simulink model "TrajectoryFollowVehicle"  (R2024b)
settings: Solver=FixedStepAuto  StartTime=0  StopTime=1000  FixedStep=timeStep  RelTol=1e-3
PostLoadFcn:
  | load(fullfile(matlabroot,'toolbox','driving','drivingdata','rrScenarioSimTypes.mat'));
  | helperSLTrajectoryFollowerWithRRScenarioSetup
undefined symbols (not defined in the file or in its folder): Defined, Ego, Lane, lr, m, n, Pose, RRtimeStep, tau, tau2, timeStep, User, Velocity
libraries: roadrunnerscenario x6, simulink_extras x6, drivingvehiclecontroller x2, autolibshared x1
settings Model: Creator=The MathWorks, Inc.  LastModifiedBy=nobuakif
settings DataIOCC: SaveOutput=off  DSMLogging=off  InspectSignalLogs=on  SaveTime=off  ReturnWorkspaceOutputs=off
settings OptimizationCC: DefaultParameterBehavior=Inlined  ReuseModelBlockBuffer=off  ZeroExternalMemoryAtStartup=off  ZeroInternalMemoryAtStartup=off
settings DebuggingCC: ParameterTunabilityLossMsg=error  UnconnectedInputMsg=warning  UnconnectedOutputMsg=warning  UnconnectedLineMsg=warning
settings ModelReferenceCC: EnableRefExpFcnMdlSchedulingChecks=on  PropagateSignalLabelsOutOfModel=off
settings RTWCC: GenCodeOnly=on  GenerateReport=on  TargetLang=C++  GPUComputeCapability=3.5
settings CodeAppCC: ForceParamTrailComments=on
settings GRTTargetCC: TargetLangStandard=C++03 (ISO)  CodeInterfacePackaging=C++ class

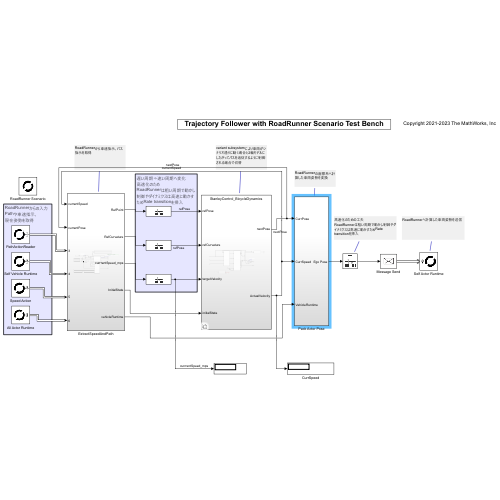
[thumbnail: Simulink's stored preview of the top-level diagram]
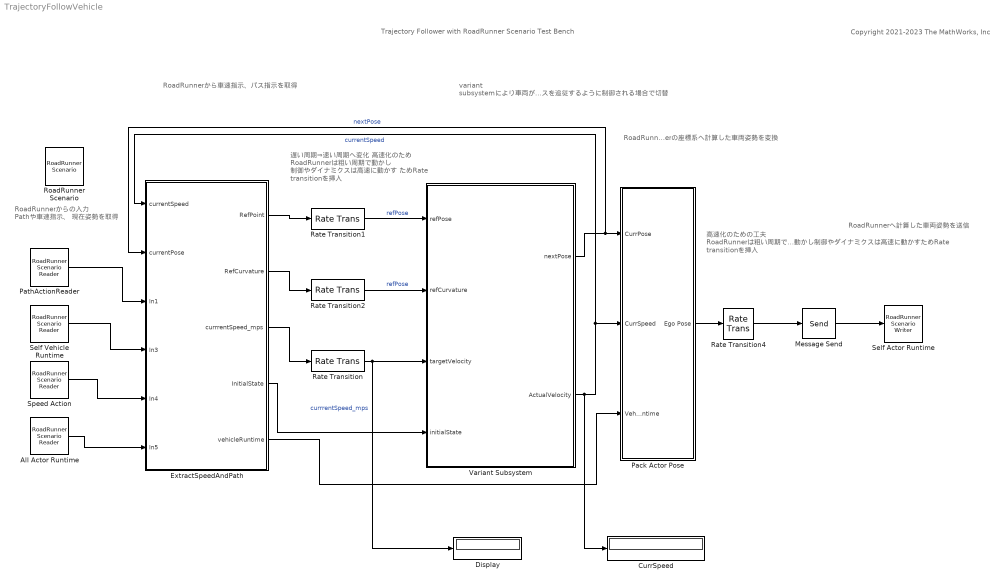
== system TrajectoryFollowVehicle ==
  note: 高速化のための工夫
      | RoadRunnerは粗い周期で動かし制御やダイナミクスは高速に動かすためRate transitionを挿入
  note: 遅い周期⇒速い周期へ変化
      | 高速化のため
      | RoadRunnerは粗い周期で動かし
      | 制御やダイナミクスは高速に動かす
      | ためRate transitionを挿入
  note: RoadRunnerからの入力
      | Pathや車速指示、
      | 現在姿勢を取得
  note: Trajectory Follower with RoadRunner Scenario Test Bench
  note: Copyright 2021-2023 The MathWorks, Inc
  note: RoadRunnerへ計算した車両姿勢を送信
  note: RoadRunnerの座標系へ計算した車両姿勢を変換
  note: variant subsystemにより車両がシナリオ通りに動く場合と2輪モデルにしたがってパスを追従するように制御される場合で切替
  note: RoadRunnerから車速指示、パス指示を取得
  All Actor Runtime : roadrunnerscenario/RoadRunner Scenario Reader  TopicCategory=Actor  ActorCategory=All Types  ActionType=Path Following  EventType=User-Defined  TopicType=Actor Pose  VehicleType=Vehicle Specifications  UserDefinedAction=Action1  UserDefinedEvent=Event1  Filter=None  SensorTopic=Target Poses  LaneBoundaryOutputTopic=Ego-Lane  SensorID=1  SampleTime=RRtimeStep
  CurrSpeed : Display
  Display : Display
  ExtractSpeedAndPath : Subsystem
  Message Send : Send  OutputPortMessageModes=m
  Pack Actor Pose : Subsystem
  PathActionReader : roadrunnerscenario/RoadRunner Scenario Reader  TopicCategory=Action  ActorCategory=Vehicle  ActionType=Path Following  EventType=User-Defined  TopicType=Actor Specifications  VehicleType=Vehicle Pose  UserDefinedAction=Action1  UserDefinedEvent=Event1  Filter=Self  SensorTopic=Target Poses  LaneBoundaryOutputTopic=Ego-Lane  SensorID=1  SampleTime=RRtimeStep
  Rate Transition : RateTransition  OutPortSampleTime=timeStep
  Rate Transition1 : RateTransition  OutPortSampleTime=timeStep
  Rate Transition2 : RateTransition  OutPortSampleTime=timeStep
  Rate Transition4 : RateTransition  OutPortSampleTime=RRtimeStep
  RoadRunner Scenario : roadrunnerscenario/RoadRunner Scenario  UserDefinedActions={}  UserDefinedEvents={}
  Self Actor Runtime : roadrunnerscenario/RoadRunner Scenario Writer  TopicCategory=Actor  ActorCategory=All Types  EventType=Action Complete  UserDefinedEvent=Event1  VehicleType=Vehicle Pose  TopicType=Actor Pose
  Self Vehicle Runtime : roadrunnerscenario/RoadRunner Scenario Reader  TopicCategory=Actor  ActorCategory=Vehicle  ActionType=Path Following  EventType=User-Defined  TopicType=Actor Specifications  VehicleType=Vehicle Pose  UserDefinedAction=Action1  UserDefinedEvent=Event1  Filter=Self  SensorTopic=Target Poses  LaneBoundaryOutputTopic=Ego-Lane  SensorID=1  SampleTime=RRtimeStep
  Speed Action : roadrunnerscenario/RoadRunner Scenario Reader  TopicCategory=Action  ActorCategory=All Types  ActionType=Speed Change  EventType=User-Defined  TopicType=Actor Specifications  VehicleType=Vehicle Specifications  UserDefinedAction=Action1  UserDefinedEvent=Event1  Filter=Self  SensorTopic=Target Poses  LaneBoundaryOutputTopic=Ego-Lane  SensorID=1  SampleTime=RRtimeStep
  Variant Subsystem : Subsystem  Variant=on
  wires:
  Rate Transition/1 -> Variant Subsystem/3(targetVelocity), Display/1  "currrentSpeed_mps"
  ExtractSpeedAndPath/5(vehicleRuntime) -> Pack Actor Pose/3(VehicleRuntime)
  Pack Actor Pose/1(Ego Pose) -> Rate Transition4/1
  Message Send/1 -> Self Actor Runtime/1
  Rate Transition4/1 -> Message Send/1
  Rate Transition1/1 -> Variant Subsystem/1(refPose)  "refPose"
  Variant Subsystem/2(ActualVelocity) -> CurrSpeed/1, ExtractSpeedAndPath/1(currentSpeed), Pack Actor Pose/2(CurrSpeed)  "currentSpeed"
  Variant Subsystem/1(nextPose) -> ExtractSpeedAndPath/2(currentPose), Pack Actor Pose/1(CurrPose)  "nextPose"
  Rate Transition2/1 -> Variant Subsystem/2(refCurvature)  "refPose"
  ExtractSpeedAndPath/4(InitialState) -> Variant Subsystem/4(initialState)
  PathActionReader/1 -> ExtractSpeedAndPath/3(In1)
  Self Vehicle Runtime/1 -> ExtractSpeedAndPath/4(In3)
  Speed Action/1 -> ExtractSpeedAndPath/5(In4)
  All Actor Runtime/1 -> ExtractSpeedAndPath/6(In5)
  ExtractSpeedAndPath/1(RefPoint) -> Rate Transition1/1
  ExtractSpeedAndPath/2(RefCurvature) -> Rate Transition2/1
  ExtractSpeedAndPath/3(currrentSpeed_mps) -> Rate Transition/1

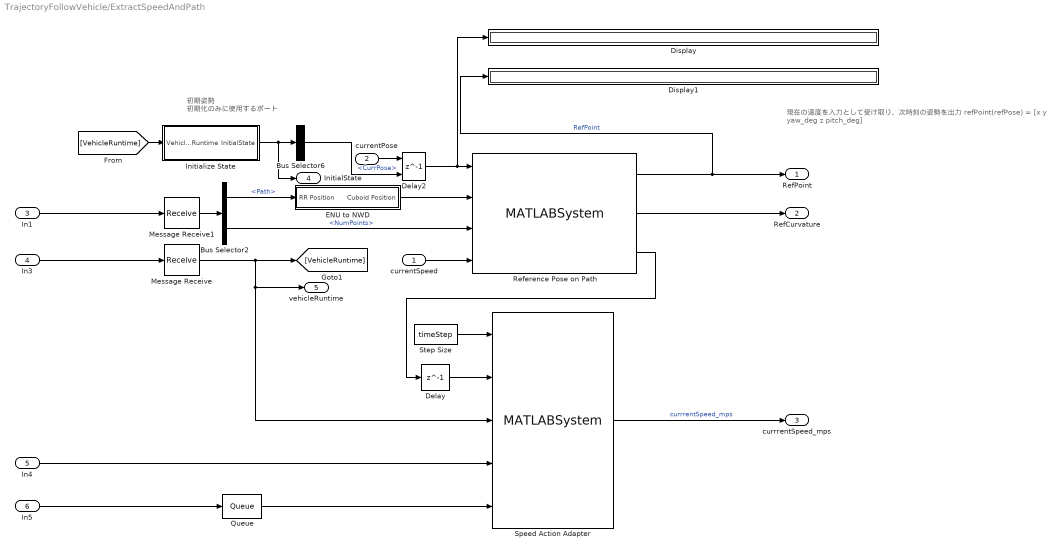
== system TrajectoryFollowVehicle/ExtractSpeedAndPath ==
  note: 現在の速度を入力として受け取り、次時刻の姿勢を出力
      | refPoint(refPose) = [x y yaw_deg z pitch_deg]
  note: 初期姿勢
      | 初期化のみに使用するポート
  currentSpeed : Inport
  currentPose : Inport  Port=2
  In1 : Inport  Port=3
  In3 : Inport  Port=4
  In4 : Inport  Port=5
  In5 : Inport  Port=6
  Bus Selector2 : BusSelector  OutputSignals=PathTarget.Path,PathTarget.NumPoints
  Bus Selector6 : BusSelector  OutputSignals=CurrPose
  Delay : Delay  DelayLength=1  InitialCondition=logical(0)
  Delay2 : Delay  DelayLength=1  InitialConditionSource=Input port
      settings: InputPortMap=u0,p4
  Display : Display
  Display1 : Display
  ENU to NWD : Subsystem
  Initialize State : Subsystem
  Message Receive : Receive  InputPortMessageModes=m
  Message Receive1 : Receive  InputPortMessageModes=m
  Queue : Queue  InputPortMessageModes=m  OutputPortMessageModes=m  OverwriteOldest=on  Capacity=16  QueueType=LIFO
  Reference Pose on Path : MATLABSystem  System=HelperReferencePoseOnPath  timeStep=timeStep  vehicleOnPath=useDynamicsStanley == false  long_offset=lf  debugFig=false  searchIndx=10
      mask Type: HelperReferencePoseOnPath
      mask Display:
      | disp(['HelperReferencePoseOnPath' char(10) '' char(10) '' char(10) '' char(10) '']);
      | port_label('input',1,'PrevVehicleInfo');
      | port_label('input',2,'Trajectory');
      | port_label('input',3,'NumTrajPoints');
      | port_label('input',4,'currentSpeed');
      | port_label('output',1,'RefPointOnPath');
      | port_label('output',2,'RefCurvature');
      | port_label('output',3,'IsGoalReached');
  Speed Action Adapter : MATLABSystem  InputPortMessageModes=n,n,n,m,m  System=HelperSpeedActionAdapter
      mask Type: HelperSpeedActionAdapter
      mask Display:
      | disp(['HelperSpeedActionAdapter' char(10) '' char(10) '']);
      | port_label('input',1,'timestep');
      | port_label('input',2,'stopVehicle');
      | port_label('input',3,'vehicleRuntime');
      | port_label('input',4,'msgSpeedAction');
      | port_label('input',5,'msgAllVehicleRuntime');
      | port_label('output',1,'currentSpeed');
  Step Size : Constant  Value=timeStep
  RefPoint : Outport
  RefCurvature : Outport  Port=2
  currrentSpeed_mps : Outport  Port=3
  InitialState : Outport  Port=4
  vehicleRuntime : Outport  Port=5
  wires:
  Bus Selector6/1 -> Delay2/2  "<CurrPose>"
  Delay/1 -> Speed Action Adapter/2
  Reference Pose on Path/1 -> Display1/1, RefPoint/1  "RefPoint"
  Step Size/1 -> Speed Action Adapter/1
  [VehicleRuntime] -> Initialize State/1(VehicleRuntime)
  Message Receive1/1 -> Bus Selector2/1
  Initialize State/1(InitialState) -> InitialState/1, Bus Selector6/1
  Reference Pose on Path/3 -> Delay/1
  Bus Selector2/1 -> ENU to NWD/1(RR Position)  "<Path>"
  Message Receive/1 -> Speed Action Adapter/3, vehicleRuntime/1, [VehicleRuntime]
  In4/1 -> Speed Action Adapter/4
  ENU to NWD/1(Cuboid Position) -> Reference Pose on Path/2
  Bus Selector2/2 -> Reference Pose on Path/3  "<NumPoints>"
  In3/1 -> Message Receive/1
  Reference Pose on Path/2 -> RefCurvature/1
  In5/1 -> Queue/1
  Speed Action Adapter/1 -> currrentSpeed_mps/1  "currrentSpeed_mps"
  In1/1 -> Message Receive1/1
  currentSpeed/1 -> Reference Pose on Path/4
  Queue/1 -> Speed Action Adapter/5
  Delay2/1 -> Display/1, Reference Pose on Path/1
  currentPose/1 -> Delay2/1

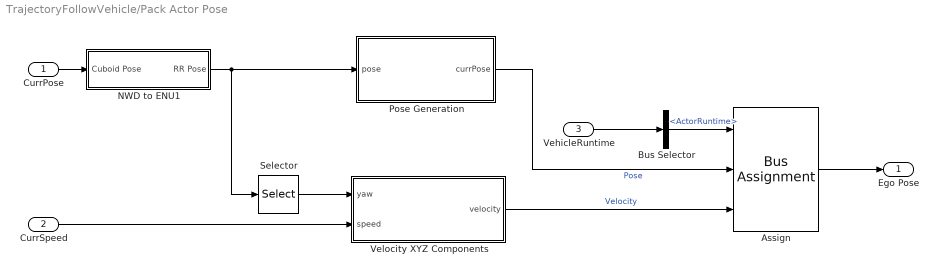
== system TrajectoryFollowVehicle/Pack Actor Pose ==
  CurrPose : Inport
  CurrSpeed : Inport  Port=2
  VehicleRuntime : Inport  Port=3
  Assign : BusAssignment  AssignedSignals=Pose,Velocity
  Bus Selector : BusSelector  OutputSignals=ActorRuntime
  NWD to ENU1 : Subsystem
  Pose Generation : MATLAB Function  TreatAsAtomicUnit=on
  Selector : Selector  InputPortWidth=5  IndexOptions=Index vector (dialog)  Indices=3  OutputSizes=1
  Velocity XYZ Components : MATLAB Function  TreatAsAtomicUnit=on
  Ego Pose : Outport
  wires:
  Velocity XYZ Components/1(velocity) -> Assign/3  "Velocity"
  Pose Generation/1(currPose) -> Assign/2  "Pose"
  CurrPose/1 -> NWD to ENU1/1(Cuboid Pose)
  Selector/1 -> Velocity XYZ Components/1(yaw)
  CurrSpeed/1 -> Velocity XYZ Components/2(speed)
  VehicleRuntime/1 -> Bus Selector/1
  Bus Selector/1 -> Assign/1  "<ActorRuntime>"
  Assign/1 -> Ego Pose/1
  NWD to ENU1/1(RR Pose) -> Selector/1, Pose Generation/1(pose)

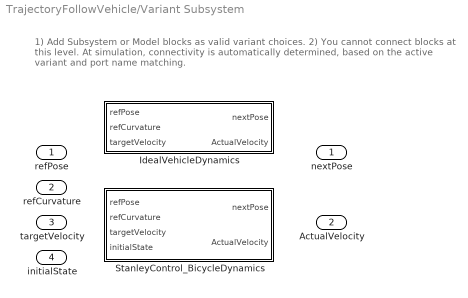
== system TrajectoryFollowVehicle/Variant Subsystem ==
  note: 1) Add Subsystem or Model blocks as valid variant choices.
      | 2) You cannot connect blocks at this level. At simulation, connectivity is automatically
      | determined, based on the active variant and port name matching.
  refPose : Inport
  refCurvature : Inport  Port=2
  targetVelocity : Inport  Port=3
  initialState : Inport  Port=4
  IdealVehicleDynamics : Subsystem  VariantControl=useDynamicsStanley == false
  StanleyControl_BicycleDynamics : Subsystem  VariantControl=useDynamicsStanley == true
  nextPose : Outport
  ActualVelocity : Outport  Port=2

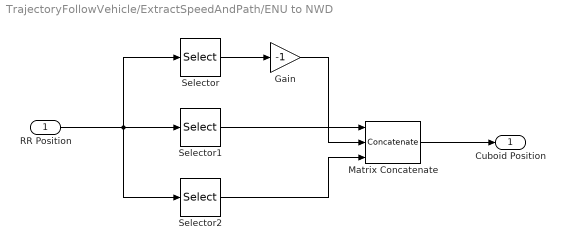
== system TrajectoryFollowVehicle/ExtractSpeedAndPath/ENU to NWD ==
  RR Position : Inport
  Gain : Gain  Gain=-1
  Matrix Concatenate : Concatenate  NumInputs=3  Mode=Multidimensional array  ConcatenateDimension=2
  Selector : Selector  NumberOfDimensions=2  InputPortWidth=3  IndexOptions=Select all,Index vector (dialog)  Indices=[1 3],1  OutputSizes=1,1
  Selector1 : Selector  NumberOfDimensions=2  InputPortWidth=3  IndexOptions=Select all,Index vector (dialog)  Indices=[1 3],2  OutputSizes=1,1
  Selector2 : Selector  NumberOfDimensions=2  InputPortWidth=3  IndexOptions=Select all,Index vector (dialog)  Indices=[1 3],3  OutputSizes=1,1
  Cuboid Position : Outport
  wires:
  Gain/1 -> Matrix Concatenate/2
  Selector1/1 -> Matrix Concatenate/1
  Selector2/1 -> Matrix Concatenate/3
  Selector/1 -> Gain/1
  RR Position/1 -> Selector/1, Selector1/1, Selector2/1
  Matrix Concatenate/1 -> Cuboid Position/1

== system TrajectoryFollowVehicle/ExtractSpeedAndPath/Initialize State ==
  VehicleRuntime : Inport
  Calculate Initial States : Subsystem
  Constant : Constant  Value=0
  Delay : Delay  DelayLength=1  InitialCondition=1
  InitialState : Outport
  wires:
  Delay/1 -> Calculate Initial States/Trigger
  Constant/1 -> Delay/1
  Calculate Initial States/1(EgoInitialState) -> InitialState/1
  VehicleRuntime/1 -> Calculate Initial States/1(EgoRuntime)

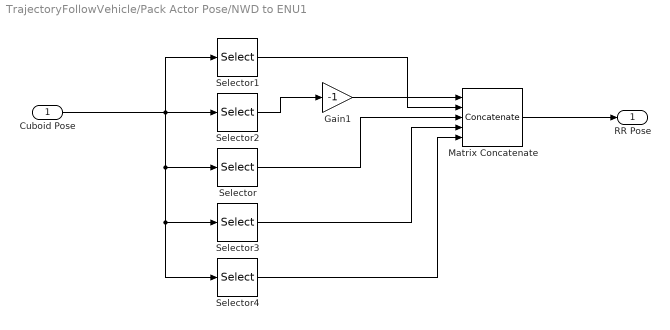
== system TrajectoryFollowVehicle/Pack Actor Pose/NWD to ENU1 ==
  Cuboid Pose : Inport
  Gain1 : Gain  Gain=-1
  Matrix Concatenate : Concatenate  NumInputs=5  Mode=Multidimensional array  ConcatenateDimension=2
  Selector : Selector  InputPortWidth=5  IndexOptions=Index vector (dialog)  Indices=3  OutputSizes=1
  Selector1 : Selector  InputPortWidth=5  IndexOptions=Index vector (dialog)  Indices=1  OutputSizes=1
  Selector2 : Selector  InputPortWidth=5  IndexOptions=Index vector (dialog)  Indices=2  OutputSizes=1
  Selector3 : Selector  InputPortWidth=5  IndexOptions=Index vector (dialog)  Indices=4  OutputSizes=1
  Selector4 : Selector  InputPortWidth=5  IndexOptions=Index vector (dialog)  Indices=5  OutputSizes=1
  RR Pose : Outport
  wires:
  Gain1/1 -> Matrix Concatenate/1
  Cuboid Pose/1 -> Selector2/1, Selector/1, Selector3/1, Selector4/1, Selector1/1
  Selector/1 -> Matrix Concatenate/3
  Selector1/1 -> Matrix Concatenate/2
  Selector2/1 -> Gain1/1
  Matrix Concatenate/1 -> RR Pose/1
  Selector3/1 -> Matrix Concatenate/4
  Selector4/1 -> Matrix Concatenate/5

== system TrajectoryFollowVehicle/Variant Subsystem/IdealVehicleDynamics ==
  refPose : Inport
  refCurvature : Inport  Port=2
  targetVelocity : Inport  Port=3
  Terminator : Terminator
  nextPose : Outport
  ActualVelocity : Outport  Port=2
  wires:
  targetVelocity/1 -> ActualVelocity/1
  refCurvature/1 -> Terminator/1
  refPose/1 -> nextPose/1

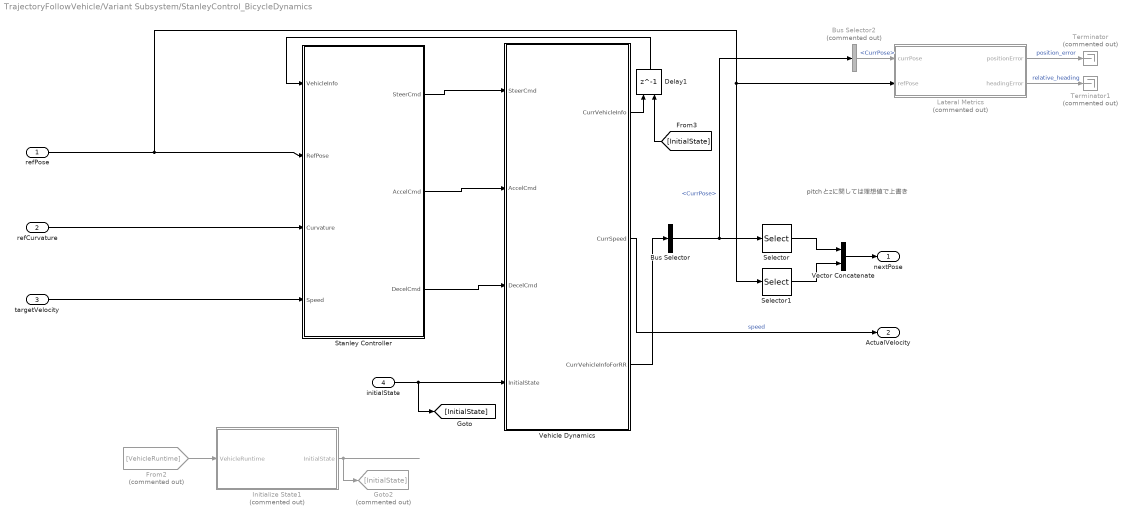
== system TrajectoryFollowVehicle/Variant Subsystem/StanleyControl_BicycleDynamics ==
  note: pitchとzに関しては理想値で上書き
  refPose : Inport
  refCurvature : Inport  Port=2
  targetVelocity : Inport  Port=3
  initialState : Inport  Port=4
  Bus Selector : BusSelector  OutputSignals=CurrPose
  Bus Selector2 : BusSelector  Commented=on  OutputSignals=CurrPose
  Delay1 : Delay  DelayLength=1  InitialConditionSource=Input port
      settings: InputPortMap=u0,p4
  From2 : From  Commented=on  GotoTag=VehicleRuntime
  Goto2 : Goto  Commented=on  GotoTag=InitialState
  Initialize State1 : Subsystem  Commented=on
  Lateral Metrics : MATLAB Function  Commented=on  TreatAsAtomicUnit=on
  Selector : Selector  InputPortWidth=5  IndexOptions=Index vector (dialog)  Indices=1:3  OutputSizes=1
  Selector1 : Selector  InputPortWidth=5  IndexOptions=Index vector (dialog)  Indices=4:5  OutputSizes=1
  Stanley Controller : Subsystem
  Terminator : Terminator  Commented=on
  Terminator1 : Terminator  Commented=on
  Vector Concatenate : Concatenate
  Vehicle Dynamics : Subsystem
  nextPose : Outport
  ActualVelocity : Outport  Port=2
  wires:
  Stanley Controller/3(DecelCmd) -> Vehicle Dynamics/3(DecelCmd)
  Vehicle Dynamics/1(CurrVehicleInfo) -> Delay1/1
  refCurvature/1 -> Stanley Controller/3(Curvature)
  Vehicle Dynamics/2(CurrSpeed) -> ActualVelocity/1  "speed"
  Delay1/1 -> Stanley Controller/1(VehicleInfo)
  Stanley Controller/1(SteerCmd) -> Vehicle Dynamics/1(SteerCmd)
  targetVelocity/1 -> Stanley Controller/4(Speed)
  Bus Selector/1 -> Bus Selector2/1, Selector/1  "<CurrPose>"
  Stanley Controller/2(AccelCmd) -> Vehicle Dynamics/2(AccelCmd)
  [InitialState] -> Delay1/2
  Initialize State1/1(InitialState) -> Goto2/1
  From2/1 -> Initialize State1/1(VehicleRuntime)
  initialState/1 -> [InitialState], Vehicle Dynamics/4(InitialState)
  Selector/1 -> Vector Concatenate/1
  Selector1/1 -> Vector Concatenate/2
  Vector Concatenate/1 -> nextPose/1
  refPose/1 -> Selector1/1, Lateral Metrics/2(refPose), Stanley Controller/2(RefPose)
  Lateral Metrics/2(headingError) -> Terminator1/1  "relative_heading"
  Bus Selector2/1 -> Lateral Metrics/1(currPose)  "<CurrPose>"
  Lateral Metrics/1(positionError) -> Terminator/1  "position_error"
  Vehicle Dynamics/3(CurrVehicleInfoForRR) -> Bus Selector/1

== system TrajectoryFollowVehicle/ExtractSpeedAndPath/Initialize State/Calculate Initial States ==
  EgoRuntime : Inport
  Trigger : TriggerPort  VariantControl=(inherit)  InitialTriggerSignalState=negative  PortDimensions=1
  Calculate Initial States : MATLAB Function  TreatAsAtomicUnit=on
  EgoInitialState : Outport
  wires:
  EgoRuntime/1 -> Calculate Initial States/1(egoRuntime)
  Calculate Initial States/1(egoInitialState) -> EgoInitialState/1

== system TrajectoryFollowVehicle/Variant Subsystem/StanleyControl_BicycleDynamics/Initialize State1 ==
  VehicleRuntime : Inport
  Calculate Initial States : Subsystem
  Constant : Constant  Value=0
  Delay : Delay  DelayLength=1  InitialCondition=1
  InitialState : Outport
  wires:
  Delay/1 -> Calculate Initial States/Trigger
  Constant/1 -> Delay/1
  Calculate Initial States/1(EgoInitialState) -> InitialState/1
  VehicleRuntime/1 -> Calculate Initial States/1(EgoRuntime)

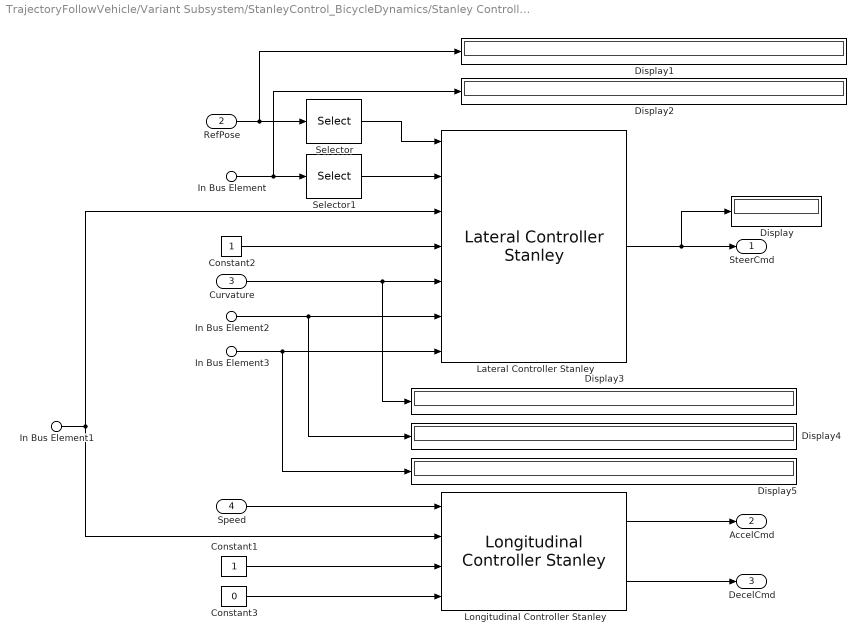
== system TrajectoryFollowVehicle/Variant Subsystem/StanleyControl_BicycleDynamics/Stanley Controller ==
  In Bus Element : Inport  PortName=VehicleInfo  Element=CurrPose
  In Bus Element1 : Inport  PortName=VehicleInfo  Element=CurrVelocity
  In Bus Element2 : Inport  PortName=VehicleInfo  Element=CurrYawRate
  In Bus Element3 : Inport  PortName=VehicleInfo  Element=CurrSteer
  RefPose : Inport  Port=2
  Curvature : Inport  Port=3
  Speed : Inport  Port=4
  Constant1 : Constant
  Constant2 : Constant
  Constant3 : Constant  Value=0
  Display{,1..5} (6 alike) : Display
  Lateral Controller Stanley : drivingvehiclecontroller/Lateral Controller Stanley  ModelType=Dynamic bicycle model  PositionGainF=3  PositionGainR=2.5  YawRateGain=0.2  DelayGain=0.2  VehicleMass=m  Lf=lf  Lr=lr  TireStiffness=Cf  Wheelbase=2.8  MaxSteeringAngle=30
  Longitudinal Controller Stanley : drivingvehiclecontroller/Longitudinal Controller Stanley  Kp=2  Ki=1  SampleTime=timeStep  MaxAcceleration=max_ac  MaxDeceleration=max_dc
  Selector : Selector  InputPortWidth=5  IndexOptions=Index vector (dialog)  Indices=[1:3]  OutputSizes=1
  Selector1 : Selector  InputPortWidth=5  IndexOptions=Index vector (dialog)  Indices=[1:3]  OutputSizes=1
  SteerCmd : Outport
  AccelCmd : Outport  Port=2
  DecelCmd : Outport  Port=3
  wires:
  In Bus Element/1 -> Display2/1, Selector1/1
  Lateral Controller Stanley/1 -> Display/1, SteerCmd/1
  In Bus Element2/1 -> Display4/1, Lateral Controller Stanley/6
  In Bus Element1/1 -> Lateral Controller Stanley/3, Longitudinal Controller Stanley/2
  Constant1/1 -> Longitudinal Controller Stanley/3
  Longitudinal Controller Stanley/2 -> DecelCmd/1
  Constant2/1 -> Lateral Controller Stanley/4
  In Bus Element3/1 -> Display5/1, Lateral Controller Stanley/7
  Constant3/1 -> Longitudinal Controller Stanley/4
  RefPose/1 -> Display1/1, Selector/1
  Longitudinal Controller Stanley/1 -> AccelCmd/1
  Curvature/1 -> Display3/1, Lateral Controller Stanley/5
  Speed/1 -> Longitudinal Controller Stanley/1
  Selector/1 -> Lateral Controller Stanley/1
  Selector1/1 -> Lateral Controller Stanley/2

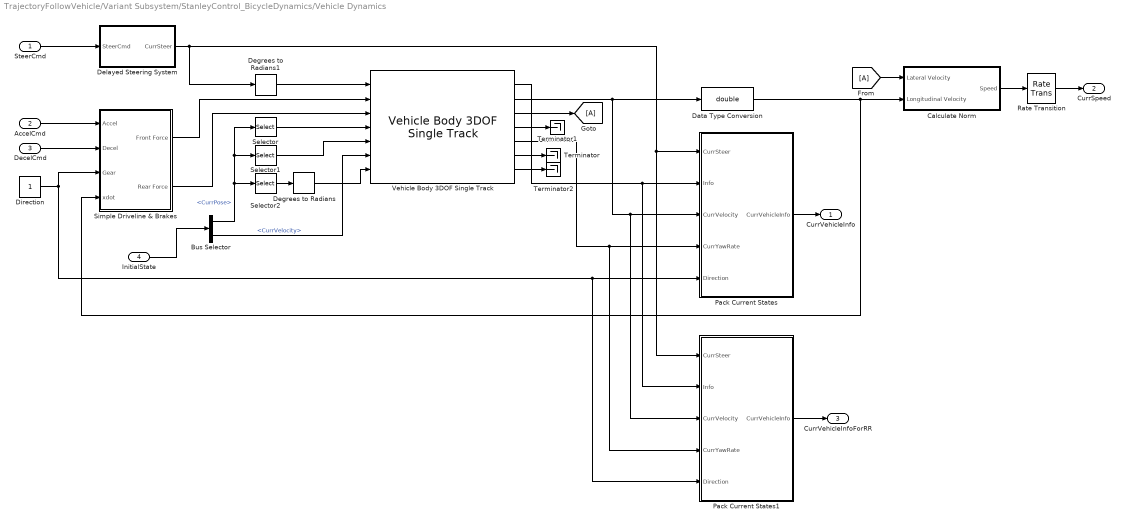
== system TrajectoryFollowVehicle/Variant Subsystem/StanleyControl_BicycleDynamics/Vehicle Dynamics ==
  SteerCmd : Inport
  AccelCmd : Inport  Port=2
  DecelCmd : Inport  Port=3
  InitialState : Inport  Port=4
  Bus Selector : BusSelector  OutputSignals=CurrPose,CurrVelocity
  Calculate Norm : Subsystem
  Data Type Conversion : DataTypeConversion  OutDataTypeStr=double  SaturateOnIntegerOverflow=off  RndMeth=Floor
  Degrees to Radians : simulink_extras/Transformations/Degrees to Radians
  Degrees to Radians1 : simulink_extras/Transformations/Degrees to Radians
  Delayed Steering System : Subsystem
  Direction : Constant
  From : From
  Goto : Goto
  Pack Current States : Subsystem
  Pack Current States1 : Subsystem
  Rate Transition : RateTransition
  Selector : Selector  InputPortWidth=5  IndexOptions=Index vector (dialog)  Indices=1  OutputSizes=1
  Selector1 : Selector  InputPortWidth=5  IndexOptions=Index vector (dialog)  Indices=2  OutputSizes=1
  Selector2 : Selector  InputPortWidth=5  IndexOptions=Index vector (dialog)  Indices=3  OutputSizes=1
  Simple Driveline & Brakes : Subsystem
  Terminator : Terminator
  Terminator1 : Terminator
  Terminator2 : Terminator
  Vehicle Body 3DOF Single Track : autolibshared/Vehicle Body 3DOF Single Track  trackMode=Single (bicycle)  inputMode=External longitudinal forces  frontSteerMode=on  rearSteerMode=off  windMode=off  muMode=off  extFMode=off  extMMode=off  htchFMode=off  htchMMode=off  extXo=on  extpsio=on  extxdoto=on  extro=off  extYo=on  extTamb=off  extydoto=off  aMode=2  NF=2  NR=2  m=m  a=lf  b=lr  h=0.35  dh=1  hh=0.2  X_o=0  xdot_o=0  CalphaMode=off  sigmaMode=off  d=0  hl=0  w=[1.4,1.4]  Cy_f=Cf  Cy_r=Cr  sigma_f=.1  sigma_r=.1  alpha_f_brk=[-.1 .1]  Cy_f_data=[-9e3 9e3]  alpha_r_brk=[-.1 .1]  Cy_r_data=[-9e3 9e3]  Y_o=0  ydot_o=0  Izz=Iz  psi_o=0  r_o=0  Af=0  Cd=.3  Cl=.1  Cpm=.1  beta_w=[0:0.01:0.3]  Cs=[0:0.03:0.9]  Cym=[0:0.01:0.3]  Pabs=101325  Tair=273  g=9.81  mu=1  xdot_tol=.01  Fznom=5000  Fxtire_sat=7e4  Fytire_sat=7e4  longOff=0  latOff=0  vertOff=0  wrapAng=off
  CurrVehicleInfo : Outport  VectorParamsAs1DForOutWhenUnconnected=off
  CurrSpeed : Outport  Port=2
  CurrVehicleInfoForRR : Outport  Port=3  VectorParamsAs1DForOutWhenUnconnected=off
  wires:
  DecelCmd/1 -> Simple Driveline & Brakes/2(Decel)
  AccelCmd/1 -> Simple Driveline & Brakes/1(Accel)
  SteerCmd/1 -> Delayed Steering System/1(SteerCmd)
  Direction/1 -> Pack Current States1/5(Direction), Pack Current States/5(Direction), Simple Driveline & Brakes/3(Gear)
  Vehicle Body 3DOF Single Track/2 -> Data Type Conversion/1, Pack Current States1/3(CurrVelocity), Pack Current States/3(CurrVelocity)
  Delayed Steering System/1(CurrSteer) -> Degrees to Radians1/1, Pack Current States1/1(CurrSteer), Pack Current States/1(CurrSteer)
  From/1 -> Calculate Norm/1(Lateral Velocity)
  Calculate Norm/1(Speed) -> Rate Transition/1
  Vehicle Body 3DOF Single Track/1 -> Pack Current States1/2(Info), Pack Current States/2(Info)
  Vehicle Body 3DOF Single Track/4 -> Terminator1/1
  Vehicle Body 3DOF Single Track/5 -> Pack Current States1/4(CurrYawRate), Pack Current States/4(CurrYawRate)
  Pack Current States/1(CurrVehicleInfo) -> CurrVehicleInfo/1
  Vehicle Body 3DOF Single Track/3 -> Goto/1
  Data Type Conversion/1 -> Calculate Norm/2(Longitudinal Velocity), Simple Driveline & Brakes/4(xdot)
  Rate Transition/1 -> CurrSpeed/1
  Vehicle Body 3DOF Single Track/7 -> Terminator2/1
  Vehicle Body 3DOF Single Track/6 -> Terminator/1
  InitialState/1 -> Bus Selector/1
  Degrees to Radians1/1 -> Vehicle Body 3DOF Single Track/1
  Simple Driveline & Brakes/1(Front Force) -> Vehicle Body 3DOF Single Track/2
  Simple Driveline & Brakes/2(Rear Force) -> Vehicle Body 3DOF Single Track/3
  Bus Selector/1 -> Selector2/1, Selector1/1, Selector/1  "<CurrPose>"
  Selector/1 -> Vehicle Body 3DOF Single Track/4
  Selector1/1 -> Vehicle Body 3DOF Single Track/5
  Selector2/1 -> Degrees to Radians/1
  Bus Selector/2 -> Vehicle Body 3DOF Single Track/6  "<CurrVelocity>"
  Degrees to Radians/1 -> Vehicle Body 3DOF Single Track/7
  Pack Current States1/1(CurrVehicleInfo) -> CurrVehicleInfoForRR/1

== system TrajectoryFollowVehicle/Variant Subsystem/StanleyControl_BicycleDynamics/Initialize State1/Calculate Initial States ==
  EgoRuntime : Inport
  Trigger : TriggerPort  VariantControl=(inherit)  InitialTriggerSignalState=negative  PortDimensions=1
  Calculate Initial States : MATLAB Function  TreatAsAtomicUnit=on
  EgoInitialState : Outport
  wires:
  EgoRuntime/1 -> Calculate Initial States/1(egoRuntime)
  Calculate Initial States/1(egoInitialState) -> EgoInitialState/1

== system TrajectoryFollowVehicle/Variant Subsystem/StanleyControl_BicycleDynamics/Vehicle Dynamics/Calculate Norm ==
  Lateral Velocity : Inport
  Longitudinal Velocity : Inport  Port=2
  Add : Sum
  Math Function : Math  Operator=square
  Math Function1 : Math  Operator=square
  Sqrt : Sqrt
  Speed : Outport
  wires:
  Add/1 -> Sqrt/1
  Math Function1/1 -> Add/2
  Math Function/1 -> Add/1
  Sqrt/1 -> Speed/1
  Lateral Velocity/1 -> Math Function/1
  Longitudinal Velocity/1 -> Math Function1/1

== system TrajectoryFollowVehicle/Variant Subsystem/StanleyControl_BicycleDynamics/Vehicle Dynamics/Delayed Steering System ==
  SteerCmd : Inport
  Add : Sum  Inputs=+-
  Delay : TransferFcn  Denominator=[0.1 0]
  Display : Display
  Display1 : Display
  Display2 : Display
  CurrSteer : Outport  VectorParamsAs1DForOutWhenUnconnected=off
  wires:
  Add/1 -> Display/1, Delay/1
  SteerCmd/1 -> Display2/1, Add/1
  Delay/1 -> Display1/1, Add/2, CurrSteer/1

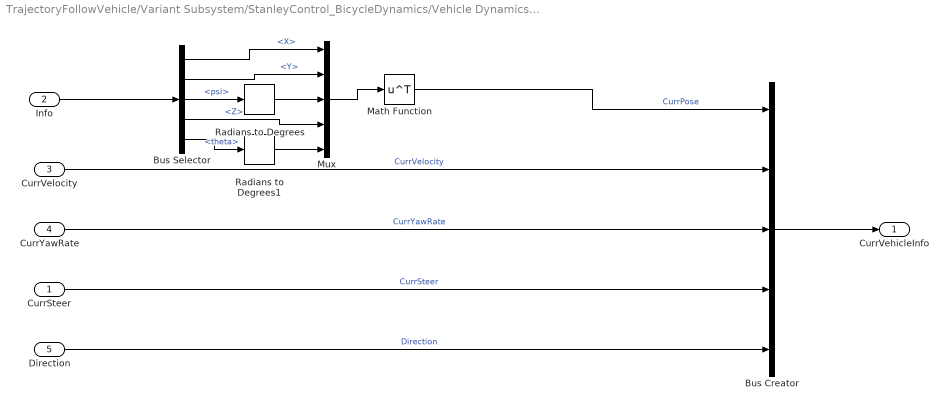
== system TrajectoryFollowVehicle/Variant Subsystem/StanleyControl_BicycleDynamics/Vehicle Dynamics/Pack Current States ==
  CurrSteer : Inport
  Info : Inport  Port=2
  CurrVelocity : Inport  Port=3
  CurrYawRate : Inport  Port=4
  Direction : Inport  Port=5
  Bus Creator : BusCreator  Inputs=5  OutDataTypeStr=Bus: BusVehicleInfo  NonVirtualBus=on
      settings: InheritFromInputs=off
  Bus Selector : BusSelector  OutputSignals=InertFrm.RearAxl.Disp.X,InertFrm.RearAxl.Disp.Y,InertFrm.Cg.Ang.psi,InertFrm.RearAxl.Disp.Z,InertFrm.Cg.Ang.theta
  Math Function : Math  Operator=transpose  SignedPower=on
  Mux : Mux  Inputs=5
  Radians to Degrees : simulink_extras/Transformations/Radians to Degrees
  Radians to Degrees1 : simulink_extras/Transformations/Radians to Degrees
  CurrVehicleInfo : Outport  VectorParamsAs1DForOutWhenUnconnected=off
  wires:
  CurrVelocity/1 -> Bus Creator/2  "CurrVelocity"
  CurrSteer/1 -> Bus Creator/4  "CurrSteer"
  Math Function/1 -> Bus Creator/1  "CurrPose"
  CurrYawRate/1 -> Bus Creator/3  "CurrYawRate"
  Direction/1 -> Bus Creator/5  "Direction"
  Mux/1 -> Math Function/1
  Info/1 -> Bus Selector/1
  Radians to Degrees/1 -> Mux/3
  Bus Selector/2 -> Mux/2  "<Y>"
  Bus Selector/1 -> Mux/1  "<X>"
  Bus Selector/3 -> Radians to Degrees/1  "<psi>"
  Bus Creator/1 -> CurrVehicleInfo/1
  Bus Selector/4 -> Mux/4  "<Z>"
  Bus Selector/5 -> Radians to Degrees1/1  "<theta>"
  Radians to Degrees1/1 -> Mux/5

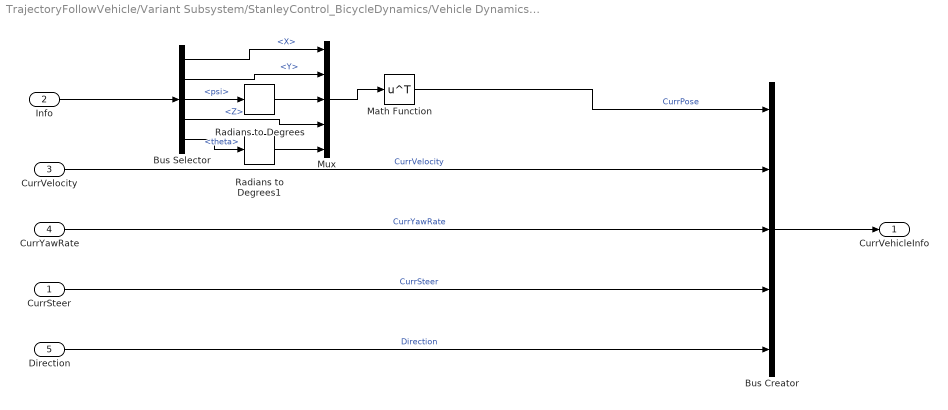
== system TrajectoryFollowVehicle/Variant Subsystem/StanleyControl_BicycleDynamics/Vehicle Dynamics/Pack Current States1 ==
  CurrSteer : Inport
  Info : Inport  Port=2
  CurrVelocity : Inport  Port=3
  CurrYawRate : Inport  Port=4
  Direction : Inport  Port=5
  Bus Creator : BusCreator  Inputs=5  OutDataTypeStr=Bus: BusVehicleInfo  NonVirtualBus=on
      settings: InheritFromInputs=off
  Bus Selector : BusSelector  OutputSignals=InertFrm.Cg.Disp.X,InertFrm.Cg.Disp.Y,InertFrm.Cg.Ang.psi,InertFrm.Cg.Disp.Z,InertFrm.Cg.Ang.theta
  Math Function : Math  Operator=transpose  SignedPower=on
  Mux : Mux  Inputs=5
  Radians to Degrees : simulink_extras/Transformations/Radians to Degrees
  Radians to Degrees1 : simulink_extras/Transformations/Radians to Degrees
  CurrVehicleInfo : Outport  VectorParamsAs1DForOutWhenUnconnected=off
  wires:
  Radians to Degrees1/1 -> Mux/5
  Bus Selector/5 -> Radians to Degrees1/1  "<theta>"
  Bus Selector/4 -> Mux/4  "<Z>"
  Bus Creator/1 -> CurrVehicleInfo/1
  Bus Selector/3 -> Radians to Degrees/1  "<psi>"
  Bus Selector/1 -> Mux/1  "<X>"
  Bus Selector/2 -> Mux/2  "<Y>"
  Radians to Degrees/1 -> Mux/3
  Info/1 -> Bus Selector/1
  Mux/1 -> Math Function/1
  Direction/1 -> Bus Creator/5  "Direction"
  CurrYawRate/1 -> Bus Creator/3  "CurrYawRate"
  Math Function/1 -> Bus Creator/1  "CurrPose"
  CurrSteer/1 -> Bus Creator/4  "CurrSteer"
  CurrVelocity/1 -> Bus Creator/2  "CurrVelocity"

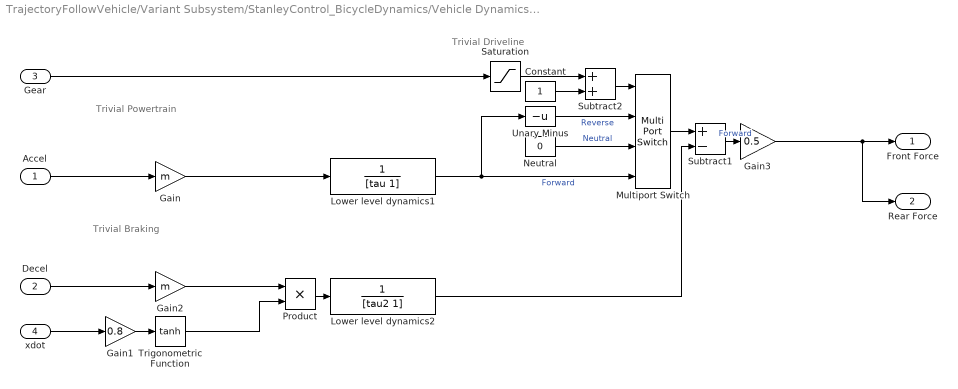
== system TrajectoryFollowVehicle/Variant Subsystem/StanleyControl_BicycleDynamics/Vehicle Dynamics/Simple Driveline & Brakes ==
  note: Trivial Driveline
  note: Trivial Powertrain
  note: Trivial Braking
  Accel : Inport
  Decel : Inport  Port=2
  Gear : Inport  Port=3
  xdot : Inport  Port=4
  Constant : Constant
  Gain : Gain  Gain=m
  Gain1 : Gain  Gain=0.8
  Gain2 : Gain  Gain=m
  Gain3 : Gain  Gain=0.5
  Lower level dynamics1 : TransferFcn  Denominator=[tau 1]
  Lower level dynamics2 : TransferFcn  Denominator=[tau2 1]
  Multiport Switch : MultiPortSwitch  DataPortOrder=Zero-based contiguous  zeroidx=on  SaturateOnIntegerOverflow=off  InputSameDT=off
  Neutral : Constant  Value=0
  Product : Product
  Saturation : Saturate  UpperLimit=1  LowerLimit=-1  ZeroCross=off
  Subtract1 : Sum  Inputs=+-
  Subtract2 : Sum
  Trigonometric Function : Trigonometry  Operator=tanh
  Unary Minus : UnaryMinus
  Front Force : Outport  VectorParamsAs1DForOutWhenUnconnected=off
  Rear Force : Outport  Port=2  VectorParamsAs1DForOutWhenUnconnected=off
  wires:
  Multiport Switch/1 -> Subtract1/1
  Accel/1 -> Gain/1
  xdot/1 -> Gain1/1
  Decel/1 -> Gain2/1
  Trigonometric Function/1 -> Product/2
  Gain1/1 -> Trigonometric Function/1
  Gain/1 -> Lower level dynamics1/1
  Gain2/1 -> Product/1
  Lower level dynamics2/1 -> Subtract1/2
  Product/1 -> Lower level dynamics2/1
  Gear/1 -> Saturation/1
  Constant/1 -> Subtract2/2
  Subtract2/1 -> Multiport Switch/1
  Neutral/1 -> Multiport Switch/3  "Neutral"
  Lower level dynamics1/1 -> Unary Minus/1, Multiport Switch/4  "Forward"
  Saturation/1 -> Subtract2/1
  Subtract1/1 -> Gain3/1  "Forward"
  Unary Minus/1 -> Multiport Switch/2  "Reverse"
  Gain3/1 -> Front Force/1, Rear Force/1

== matlab function TrajectoryFollowVehicle/Pack Actor Pose/Pose Generation ==
  data: pose input; currPose output
function currPose = generatePose(pose)
% pose = [x y yaw_rad z pitch_rad]
yaw = deg2rad(pose(3));
pitch = deg2rad(pose(5));
rotm = eul2rotm([yaw 0 pitch], "ZYX");

currPose = [[rotm [pose([1 2 4])]']; [0 0 0 1]];

== matlab function TrajectoryFollowVehicle/Variant Subsystem/StanleyControl_BicycleDynamics/Initialize State1/Calculate Initial States/Calculate Initial States ==
  data: egoRuntime input; egoInitialState output Bus: BusVehicleInfo
function egoInitialState = getInitialState(egoRuntime)
%getInitialState calculates initial conditions of the vehicle

% Calculate velocity
velocity = norm(egoRuntime.ActorRuntime.Velocity,2);
% Get Transformation matrix
transformationMatrix = egoRuntime.ActorRuntime.Pose;
% Get pose information
x = transformationMatrix(1,4);
y = transformationMatrix(2,4);
yaw = atan2d(-transformationMatrix(1,2), ...
            transformationMatrix(1,1));
z = transformationMatrix(3,4);
% pitch = atan2d(-transformationMatrix(1,2), ...
%             transformationMatrix(1,1));
pitch = 0;
% Pack the initial states CurrPose = [x y yaw_deg z pitch_deg]
egoInitialState = struct('CurrPose', [y, -x, yaw, z, pitch], ...
    'CurrVelocity', velocity, ...
    'CurrYawRate', 0, ...
    'CurrSteer',0, ...
    'Direction',1);

== matlab function TrajectoryFollowVehicle/Pack Actor Pose/Velocity XYZ Components ==
  data: yaw input size=1; velocity output size=[1 3]; speed input size=1
function velocity = computeVelocity(yaw, speed)

% Output velocity vector (x,y,z)
velocity = speed * [-sind(yaw) cosd(yaw) 0];

== matlab function TrajectoryFollowVehicle/Variant Subsystem/StanleyControl_BicycleDynamics/Lateral Metrics ==
  data: currPose input size=[1 3]; refPose input size=[1 3]; positionError output; headingError output
function [positionError, headingError] = lateralMetrics(currPose, refPose)
%lateralMetrics calculates lateral error and heading error of the vehicle 
% using current and reference pose

currPose(:,3) = deg2rad(currPose(:,3));
refPose(:,3)  = deg2rad(refPose(:,3));

positionError = norm(currPose(1:2) - refPose(1:2));

headingError = rad2deg(currPose(:, 3) - refPose(:,3));

== matlab function TrajectoryFollowVehicle/ExtractSpeedAndPath/Initialize State/Calculate Initial States/Calculate Initial States ==
  data: egoRuntime input; egoInitialState output Bus: BusVehicleInfo
function egoInitialState = getInitialState(egoRuntime)
%getInitialState calculates initial conditions of the vehicle

% Calculate velocity
velocity = norm(egoRuntime.ActorRuntime.Velocity,2);
% Get Transformation matrix
transformationMatrix = egoRuntime.ActorRuntime.Pose;
% Get pose information
x = transformationMatrix(1,4);
y = transformationMatrix(2,4);
yaw = atan2d(-transformationMatrix(1,2), ...
            transformationMatrix(1,1));
z = transformationMatrix(3,4);
eulZYX = tform2eul(transformationMatrix, "ZYX");

% yaw = eulZYX(1);
pitch = asind(transformationMatrix(2, 3));

% Pack the initial states
egoInitialState = struct('CurrPose', [y, -x, yaw, z, pitch], ...
    'CurrVelocity', velocity, ...
    'CurrYawRate', 0, ...
    'CurrSteer',0, ...
    'Direction',1);
